simulink model "controller_test"  (R2021a)
settings: Solver=ode15s  StartTime=0.0  StopTime=0.75  FixedStep=0.00001  RelTol=1
InitFcn:
  | p_init;
  | p_init_wrist;
values from neighbouring files (symbols this model uses):
  a = 0    [p_init.m]
  a_w = 0    [p_init_wrist.m]
  b = 1/1.34e6    (= 7.46268656716e-07)    [p_init.m]
  b_w = 1/1.34e6    (= 7.46268656716e-07)    [p_init_wrist.m]
  comp_time = 0.000679456 * 1.25    (= 0.00084932)    [p_init.m]
  D_m = 0.00    (= 0)    [p_init.m]
  D_w = 0.00    (= 0)    [p_init_wrist.m]
  enc_res = 0.875 * pi/180    (= 0.015271630955)    [p_init.m]
  gear_ratio = 35    [p_init.m]
  gear_ratio_w = 36    [p_init_wrist.m]
  I_m = 0.00    (= 0)    [p_init.m]
  I_w = 0    [p_init_wrist.m]
  K_b = 1/(327*2*pi/60)    (= 0.0292027418517)    [p_init.m]
  K_b_w = 1/(1100*2*pi/60)    (= 0.0086811787141)    [p_init_wrist.m]
  K_m = 29.2 / 1000    (= 0.0292)    [p_init.m]
  K_m_w = 8.71 / 1000    (= 0.00871)    [p_init_wrist.m]
  K_p = 4.72e6/1.34e6    (= 3.5223880597)    [p_init.m]
  K_p_w = 4.72e6/1.34e6    (= 3.5223880597)    [p_init_wrist.m]
  L_term = 1.61 / 1000    (= 0.00161)    [p_init.m]
  L_term_w = 0.276 / 1000    (= 0.000276)    [p_init_wrist.m]
  P_m = 2.84    [p_init.m]
  P_w = 0.55    [p_init_wrist.m]
  R_term = 37.1    [p_init.m]
  R_term_w = 92.2    [p_init_wrist.m]
  v_max_amp = +V_nom    (= 24)    [p_init.m]
  v_max_amp_w = +V_nom_w    (= 12)    [p_init_wrist.m]
  v_min_amp = -V_nom    (= -24)    [p_init.m]
  v_min_amp_w = -V_nom_w    (= -12)    [p_init_wrist.m]
undefined symbols (not defined in the file or in its folder): f, fwd_kin_vect
libraries: simulink x6, pid_lib x3, instrumentlib x2
settings Model: Creator=Konstantin  LastModifiedBy=kossio
settings SolverCC: MaxOrder=3  ZeroCrossControl=DisableAll  AlgebraicLoopSolver=TrustRegion
settings DebuggingCC: SFMachineParentedDataDiag=warning

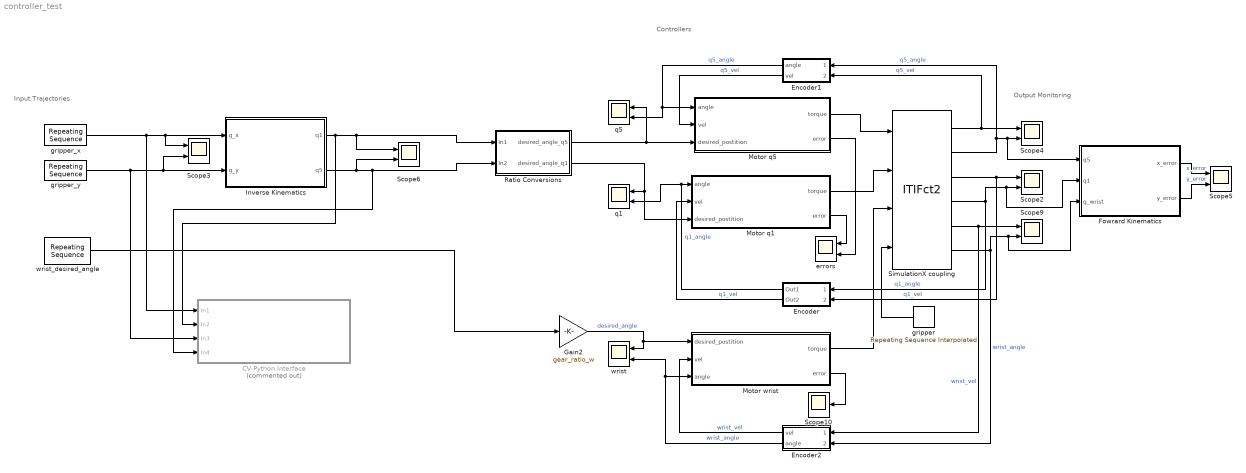
== system controller_test ==
  note: Output Monitoring
  note: Controllers
  note: Input Trajectories
  CV-Python Interface : Subsystem  Commented=on
  Encoder : Subsystem
  Encoder1 : Subsystem
  Encoder2 : Subsystem
  Fowrard Kinematics : Subsystem
  Gain2 : Gain  Gain=gear_ratio_w
  Inverse Kinematics : MATLAB Function  TreatAsAtomicUnit=on
  Motor q1 : Subsystem
  Motor q5 : Subsystem
  Motor wrist : Subsystem
  Ratio Conversions : Subsystem
  Scope10 : Scope
  Scope{2..6,9} (6 alike) : Scope  NumInputPorts=2
  SimulationX coupling : S-Function  FunctionName=ITIFct2  Parameters=ip, port, ts, nIn, nOut  SFunctionDeploymentMode=off  EnableBusSupport=off  mask{ip='localhost', port=4099, ts=0.001, nIn=4, nOut=6}
      mask prompts: ip "Address: ip"; port "Port Number: port [-]"; ts "Communication Step Size: ts [s]"; nIn "Input Vector Dimension (to SimulationX): nIn [-]"; nOut "Output Vector Dimension (from SimulationX): nOut [-]"
      mask help: Coupling Element
  errors : Scope  NumInputPorts=2
  gripper : simulink/Sources/Repeating Sequence Interpolated  OutValues=[0.2 0.2 10 0.2 10 0.2 10 0.2 0.2].'  TimeValues=[0 0.01 0.12 0.23 0.36 0.5 0.6 0.73 0.75].'  LookUpMeth=Use Input Below  tsamp=0.01  OutMin=[]  OutMax=[]  OutDataTypeStr=double  OutputDataTypeScalingMode=double  OutDataType=fixdt(0,8)  OutScaling=2^-10
  gripper_x : simulink/Sources/Repeating Sequence  rep_seq_t=time_vect  rep_seq_y=x_vect
  gripper_y : simulink/Sources/Repeating Sequence  rep_seq_t=time_vect  rep_seq_y=y_vect
  q1 : Scope  NumInputPorts=2
  q5 : Scope  NumInputPorts=2
  wrist : Scope  NumInputPorts=2
  wrist_desired_angle : simulink/Sources/Repeating Sequence  rep_seq_t=time_vect  rep_seq_y=wrist_angle
  wires:
  Inverse Kinematics/1(q1) -> CV-Python Interface/2(In2), Ratio Conversions/1(In1), Scope6/1
  Inverse Kinematics/2(q5) -> Scope6/2, Ratio Conversions/2(In2), CV-Python Interface/4(In4)
  gripper_y/1 -> CV-Python Interface/3(In3), Scope3/2, Inverse Kinematics/2(g_y)
  gripper_x/1 -> CV-Python Interface/1(In1), Inverse Kinematics/1(g_x), Scope3/1
  SimulationX coupling/1 -> Encoder1/2(2), Scope4/1  "q5_vel"
  SimulationX coupling/2 -> Fowrard Kinematics/1(q5), Scope4/2, Encoder1/1(1)  "q5_angle"
  SimulationX coupling/3 -> Encoder/2(2), Scope2/1  "q1_vel"
  SimulationX coupling/4 -> Encoder/1(1), Fowrard Kinematics/2(q1), Scope2/2  "q1_angle"
  Motor q1/2(error) -> errors/1
  Motor q5/2(error) -> errors/2
  SimulationX coupling/5 -> Encoder2/1(1), Scope9/1  "wrist_vel"
  SimulationX coupling/6 -> Fowrard Kinematics/3(q_wrist), Scope9/2, Encoder2/2(2)  "wrist_angle"
  Motor wrist/2(error) -> Scope10/1
  Motor wrist/1(torque) -> SimulationX coupling/3
  Gain2/1 -> wrist/1, Motor wrist/1(desired_postition)  "desired_angle"
  Motor q5/1(torque) -> SimulationX coupling/1
  Motor q1/1(torque) -> SimulationX coupling/2
  Encoder/1(Out1) -> q1/2, Motor q1/1(angle)  "q1_angle"
  Encoder/2(Out2) -> Motor q1/2(vel)  "q1_vel"
  Encoder1/1(angle) -> q5/2, Motor q5/1(angle)  "q5_angle"
  Encoder1/2(vel) -> Motor q5/2(vel)  "q5_vel"
  Ratio Conversions/2(desired_angle_q1) -> Motor q1/3(desired_postition), q1/1
  Ratio Conversions/1(desired_angle_q5) -> q5/1, Motor q5/3(desired_postition)
  Fowrard Kinematics/2(y_error) -> Scope5/2  "y_error"
  Fowrard Kinematics/1(x_error) -> Scope5/1  "x_error"
  wrist_desired_angle/1 -> Gain2/1
  Encoder2/1(vel) -> Motor wrist/2(vel)  "wrist_vel"
  Encoder2/2(angle) -> Motor wrist/3(angle), wrist/2  "wrist_angle"
  gripper/1 -> SimulationX coupling/4

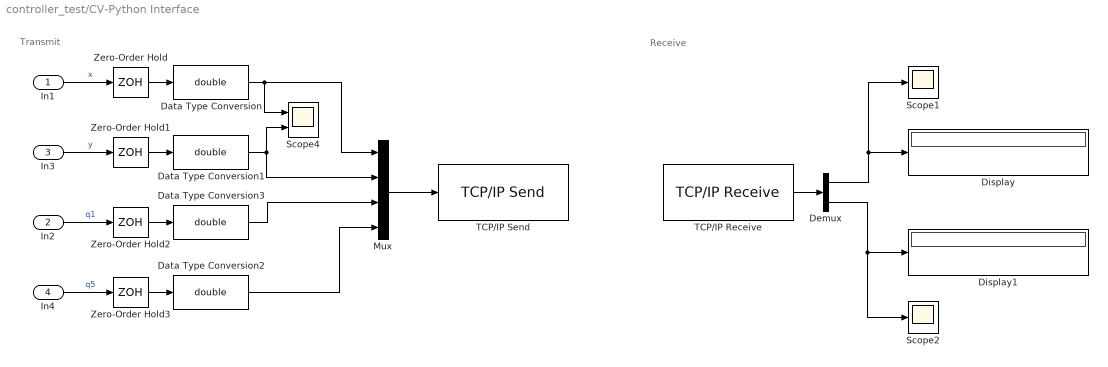
== system controller_test/CV-Python Interface ==
  note: Transmit
  note: Receive
  In1 : Inport
  In2 : Inport  Port=2
  In3 : Inport  Port=3
  In4 : Inport  Port=4
  Data Type Conversion{,1..3} (4 alike) : DataTypeConversion  OutDataTypeStr=double
  Demux : Demux  Outputs=2
  Display : Display
      settings: Format=decimal (Stored Integer)
  Display1 : Display
      settings: Format=decimal (Stored Integer)
  Mux : Mux
  Scope1 : Scope
  Scope2 : Scope
  Scope4 : Scope  NumInputPorts=2
  TCP/IP Receive : instrumentlib/TCP//IP Receive  Priority=1  Host=192.168.50.118  Port=10100  DataSize="[2  1]"  EnableBlockingMode=on  Timeout=10  SampleTime=0.01  DataType=double  ByteOrder=BigEndian  ASCIIFormatting=%f,  Terminator=LF
  TCP/IP Send : instrumentlib/TCP//IP Send  Priority=2  Host=192.168.50.118  Port=10100  EnableBlockingMode=on  Timeout=10  ByteOrder=BigEndian  TransferDelay=on
  Zero-Order Hold{,1..3} (4 alike) : ZeroOrderHold  SampleTime=0.01
  wires:
  Zero-Order Hold/1 -> Data Type Conversion/1
  TCP/IP Receive/1 -> Demux/1
  Demux/2 -> Scope2/1, Display1/1
  Zero-Order Hold2/1 -> Data Type Conversion3/1
  Data Type Conversion1/1 -> Scope4/2, Mux/2
  Zero-Order Hold1/1 -> Data Type Conversion1/1
  Demux/1 -> Display/1, Scope1/1
  Mux/1 -> TCP/IP Send/1
  Zero-Order Hold3/1 -> Data Type Conversion2/1
  Data Type Conversion/1 -> Scope4/1, Mux/1
  Data Type Conversion3/1 -> Mux/3
  Data Type Conversion2/1 -> Mux/4
  In4/1 -> Zero-Order Hold3/1  "q5"
  In2/1 -> Zero-Order Hold2/1  "q1"
  In1/1 -> Zero-Order Hold/1  "x"
  In3/1 -> Zero-Order Hold1/1  "y"

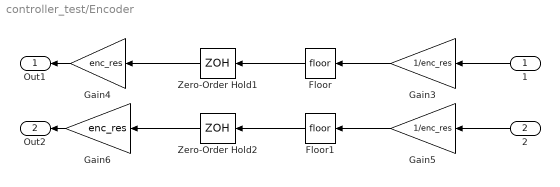
== system controller_test/Encoder ==
  1 : Inport
  2 : Inport  Port=2
  Floor : Rounding
  Floor1 : Rounding
  Gain3 : Gain  Gain=1/enc_res
  Gain4 : Gain  Gain=enc_res
  Gain5 : Gain  Gain=1/enc_res
  Gain6 : Gain  Gain=enc_res
  Zero-Order Hold1 : ZeroOrderHold  SampleTime=0.001
  Zero-Order Hold2 : ZeroOrderHold  SampleTime=0.001
  Out1 : Outport
  Out2 : Outport  Port=2
  wires:
  Zero-Order Hold2/1 -> Gain6/1
  Floor/1 -> Zero-Order Hold1/1
  Gain4/1 -> Out1/1
  Floor1/1 -> Zero-Order Hold2/1
  Gain6/1 -> Out2/1
  Gain5/1 -> Floor1/1
  Zero-Order Hold1/1 -> Gain4/1
  Gain3/1 -> Floor/1
  1/1 -> Gain3/1
  2/1 -> Gain5/1

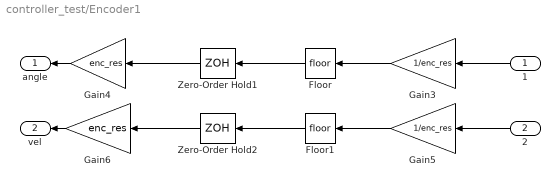
== system controller_test/Encoder1 ==
  1 : Inport
  2 : Inport  Port=2
  Floor : Rounding
  Floor1 : Rounding
  Gain3 : Gain  Gain=1/enc_res
  Gain4 : Gain  Gain=enc_res
  Gain5 : Gain  Gain=1/enc_res
  Gain6 : Gain  Gain=enc_res
  Zero-Order Hold1 : ZeroOrderHold  SampleTime=0.001
  Zero-Order Hold2 : ZeroOrderHold  SampleTime=0.001
  angle : Outport
  vel : Outport  Port=2
  wires:
  Zero-Order Hold2/1 -> Gain6/1
  Floor/1 -> Zero-Order Hold1/1
  Gain4/1 -> angle/1
  Floor1/1 -> Zero-Order Hold2/1
  Gain6/1 -> vel/1
  Gain5/1 -> Floor1/1
  Zero-Order Hold1/1 -> Gain4/1
  Gain3/1 -> Floor/1
  1/1 -> Gain3/1
  2/1 -> Gain5/1

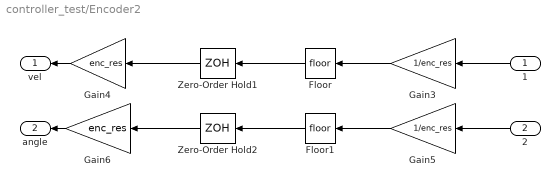
== system controller_test/Encoder2 ==
  1 : Inport
  2 : Inport  Port=2
  Floor : Rounding
  Floor1 : Rounding
  Gain3 : Gain  Gain=1/enc_res
  Gain4 : Gain  Gain=enc_res
  Gain5 : Gain  Gain=1/enc_res
  Gain6 : Gain  Gain=enc_res
  Zero-Order Hold1 : ZeroOrderHold  SampleTime=0.001
  Zero-Order Hold2 : ZeroOrderHold  SampleTime=0.001
  vel : Outport
  angle : Outport  Port=2
  wires:
  Zero-Order Hold2/1 -> Gain6/1
  Floor/1 -> Zero-Order Hold1/1
  Gain4/1 -> vel/1
  Floor1/1 -> Zero-Order Hold2/1
  Gain6/1 -> angle/1
  Gain5/1 -> Floor1/1
  Zero-Order Hold1/1 -> Gain4/1
  Gain3/1 -> Floor/1
  1/1 -> Gain3/1
  2/1 -> Gain5/1

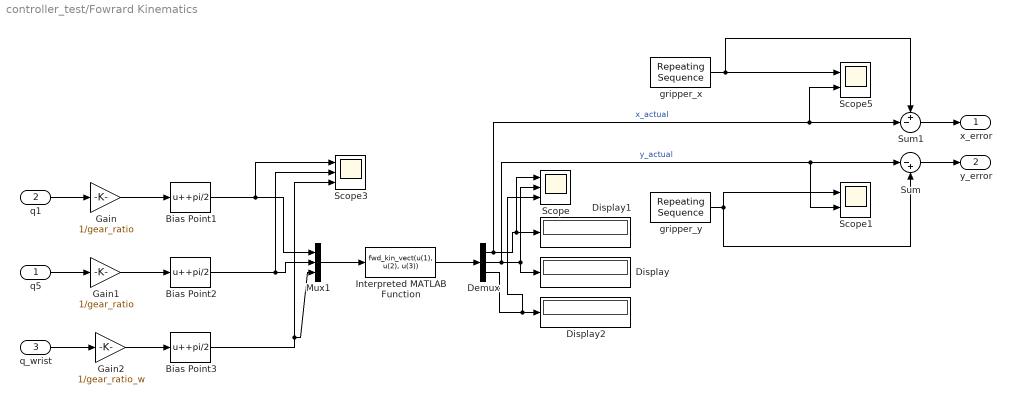
== system controller_test/Fowrard Kinematics ==
  q5 : Inport
  q1 : Inport  Port=2
  q_wrist : Inport  Port=3
  Bias Point1 : Bias  Bias=+pi/2
  Bias Point2 : Bias  Bias=+pi/2
  Bias Point3 : Bias  Bias=+pi/2
  Demux : Demux  Outputs=3
  Display : Display
  Display1 : Display
  Display2 : Display
  Gain : Gain  Gain=1/gear_ratio
  Gain1 : Gain  Gain=1/gear_ratio
  Gain2 : Gain  Gain=1/gear_ratio_w
  Interpreted MATLAB Function : MATLABFcn  MATLABFcn=fwd_kin_vect(u(1), u(2), u(3))  OutputDimensions=3
  Mux1 : Mux  Inputs=3
  Scope : Scope  NumInputPorts=3
  Scope1 : Scope  NumInputPorts=2
  Scope3 : Scope  NumInputPorts=3
  Scope5 : Scope  NumInputPorts=2
  Sum : Sum  Inputs=|-+
  Sum1 : Sum  Inputs=+-|
  gripper_x : simulink/Sources/Repeating Sequence  rep_seq_t=time_vect  rep_seq_y=x_vect
  gripper_y : simulink/Sources/Repeating Sequence  rep_seq_t=time_vect  rep_seq_y=y_vect
  x_error : Outport
  y_error : Outport  Port=2
  wires:
  Demux/3 -> Scope/3, Display2/1
  Interpreted MATLAB Function/1 -> Demux/1
  q5/1 -> Gain1/1
  Mux1/1 -> Interpreted MATLAB Function/1
  Demux/2 -> Scope1/2, Sum/1, Scope/2, Display/1  "y_actual"
  q1/1 -> Gain/1
  Demux/1 -> Scope5/2, Sum1/2, Scope/1, Display1/1  "x_actual"
  Gain/1 -> Bias Point1/1
  Gain1/1 -> Bias Point2/1
  gripper_y/1 -> Scope1/1, Sum/2
  gripper_x/1 -> Scope5/1, Sum1/1
  q_wrist/1 -> Gain2/1
  Gain2/1 -> Bias Point3/1
  Sum/1 -> y_error/1
  Sum1/1 -> x_error/1
  Bias Point1/1 -> Scope3/1, Mux1/1
  Bias Point2/1 -> Mux1/2, Scope3/2
  Bias Point3/1 -> Scope3/3, Mux1/3

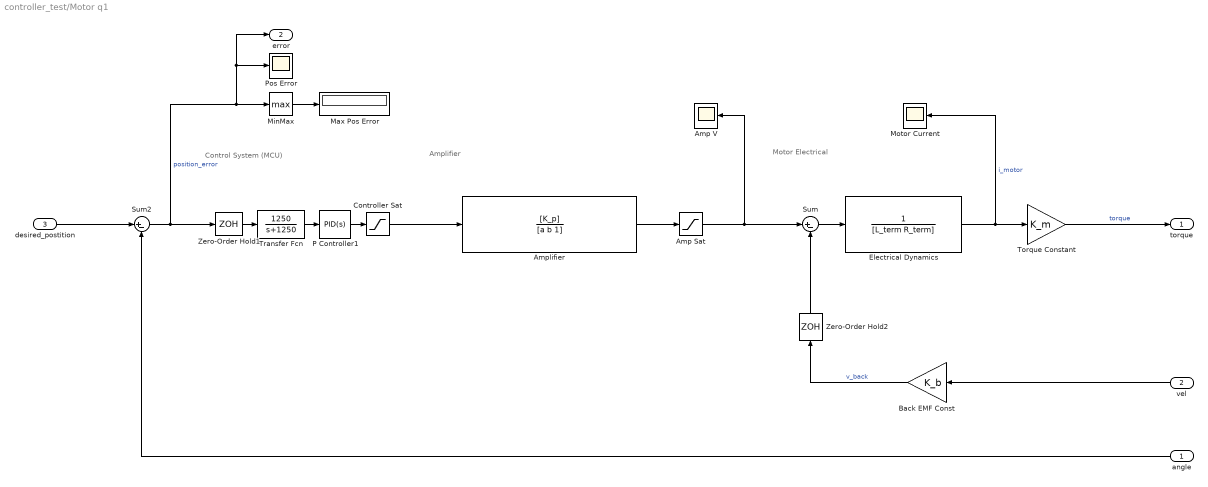
== system controller_test/Motor q1 ==
  note: Control System (MCU)
  note: Motor Electrical
  note: Amplifier
  angle : Inport
  vel : Inport  Port=2
  desired_postition : Inport  Port=3
  Amp Sat : Saturate  UpperLimit=v_max_amp  LowerLimit=v_min_amp
  Amp V : Scope
  Amplifier : TransferFcn  Numerator=[K_p]  Denominator=[a b 1]
  Back EMF Const : Gain  Gain=K_b
  Controller Sat : Saturate  UpperLimit=10  LowerLimit=-10
  Electrical Dynamics : TransferFcn  Denominator=[L_term R_term]
  Max Pos Error : Display
  MinMax : MinMax  Function=max
  Motor Current : Scope
  P Controller1 : pid_lib/PID Controller  Controller=PID  Form=Parallel  TimeDomain=Continuous-time  UseExternalTs=off  SampleTime=-1  IntegratorMethod=Forward Euler  FilterMethod=Forward Euler  ControllerParametersSource=internal  P=P_m  I=I_m  D=D_m  UseFilter=on  N=100  TunerSelectOption=Transfer Function Based (PID Tuner App)  InitialConditionSource=internal  InitialConditionForIntegrator=0  InitialConditionForFilter=0  DifferentiatorICPrevScaledInput=0  ExternalReset=none  TrackingMode=off  Kt=1  LimitOutput=off  SatLimitsSource=internal  UpperSaturationLimit=inf  LowerSaturationLimit=-inf  LinearizeAsGain=on  AntiWindupMode=none  Kb=1  POutMin=[]  POutMax=[]  IOutMin=[]  IOutMax=[]  DOutMin=[]  DOutMax=[]  NOutMin=[]  NOutMax=[]  SumOutMin=[]  SumOutMax=[]  SaturationOutMin=[]  SaturationOutMax=[]  PParamMin=[]  PParamMax=[]  IParamMin=[]  IParamMax=[]  DParamMin=[]  DParamMax=[]  NParamMin=[]  NParamMax=[]  KbParamMin=[]  KbParamMax=[]  KtParamMin=[]  KtParamMax=[]  KbOutMin=[]  KbOutMax=[]  KtOutMin=[]  KtOutMax=[]  IntegratorOutMin=[]  IntegratorOutMax=[]  FilterOutMin=[]  FilterOutMax=[]  SumI1OutMin=[]  SumI1OutMax=[]  SumI2OutMin=[]  SumI2OutMax=[]  SumI3OutMin=[]  SumI3OutMax=[]  SumI4OutMin=[]  SumI4OutMax=[]  SumDOutMin=[]  SumDOutMax=[]  DifferentiatorOutMin=[]  DifferentiatorOutMax=[]  FilterDiffOutCoefMin=[]  FilterDiffOutCoefMax=[]  ReciprocalOutMin=[]  ReciprocalOutMax=[]  SumDenOutMin=[]  SumDenOutMax=[]  SumNumOutMin=[]  SumNumOutMax=[]  DivideOutMin=[]  DivideOutMax=[]  UdiffTsProdOutMin=[]  UdiffTsProdOutMax=[]  NTsProdOutMin=[]  NTsProdOutMax=[]  UintegralTsProdOutMin=[]  UintegralTsProdOutMax=[]  UngainTsProdOutMin=[]  UngainTsProdOutMax=[]  IntegratorContinuousStateAttributes=''  IntegratorStateMustResolveToSignalObject=off  IntegratorRTWStateStorageClass=Auto  FilterContinuousStateAttributes=''  FilterStateMustResolveToSignalObject=off  FilterRTWStateStorageClass=Auto  ParallelPVariant=InternalParameters  IdealPVariant=Disabled  IVariant=InternalParameters  DVariant=InternalParameters  IntegratorVariant=Continuous  SatVariant=Disabled  AWVariant=Passthrough  PCopyVariant=Disabled  TRVariant=Disabled  FdbkBlocksVariant=Forward  IdealPFdbkVariant=Disabled  SatFdbkVariant=Disabled  DerivativeFilterVariant=ContFilter  NVariant=InternalParameters  NCopyVariant=Disabled  FilterICVariant=InternalICsFilter  IntegratorICVariant=InternalICs  ExternalResetVariant=Disabled  TRSumVariant=Passthrough  SumFdbkVariant=Disabled  SumVariant=Sum_PID  TsampFilterVariant=InternalTs  TsampNgainVariant=Passthrough  TsampIntegralVariant=Passthrough  ExternalSaturationOutDataTypeStr=Inherit: Same as second input
  Pos Error : Scope
  Sum : Sum  Inputs=|+-
  Sum2 : Sum  Inputs=|+-
  Torque Constant : Gain  Gain=K_m
  Transfer Fcn : TransferFcn  Numerator=[1250]  Denominator=[1 1250]
  Zero-Order Hold1 : ZeroOrderHold  SampleTime=comp_time
  Zero-Order Hold2 : ZeroOrderHold  SampleTime=comp_time
  torque : Outport
  error : Outport  Port=2
  wires:
  Sum2/1 -> Zero-Order Hold1/1, Pos Error/1, error/1, MinMax/1  "position_error"
  Amplifier/1 -> Amp Sat/1
  Amp Sat/1 -> Sum/1, Amp V/1
  P Controller1/1 -> Controller Sat/1
  Back EMF Const/1 -> Zero-Order Hold2/1  "v_back"
  Sum/1 -> Electrical Dynamics/1
  Electrical Dynamics/1 -> Motor Current/1, Torque Constant/1  "i_motor"
  Controller Sat/1 -> Amplifier/1
  MinMax/1 -> Max Pos Error/1
  Torque Constant/1 -> torque/1  "torque"
  angle/1 -> Sum2/2
  desired_postition/1 -> Sum2/1
  Zero-Order Hold1/1 -> Transfer Fcn/1
  vel/1 -> Back EMF Const/1
  Zero-Order Hold2/1 -> Sum/2
  Transfer Fcn/1 -> P Controller1/1

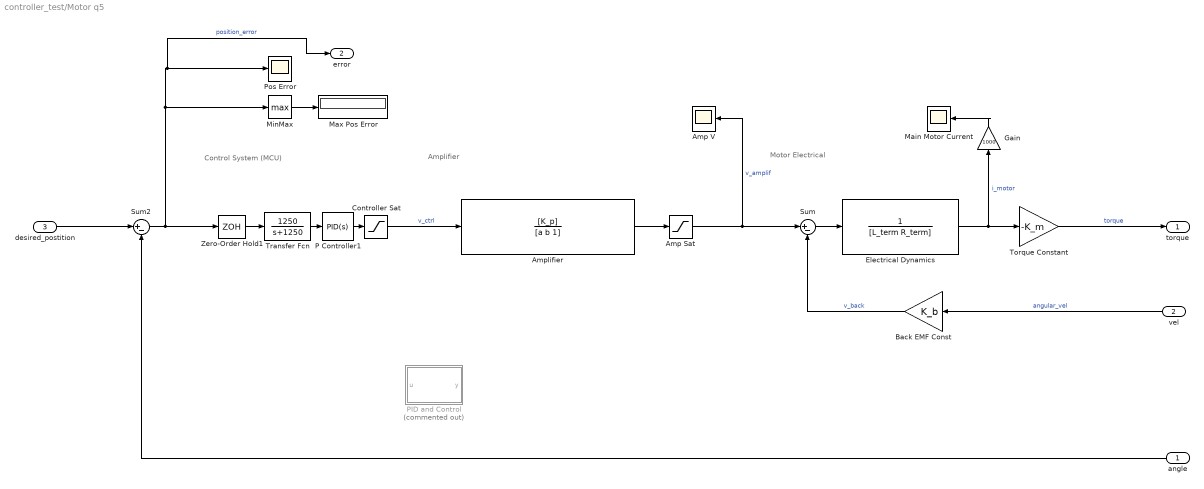
== system controller_test/Motor q5 ==
  note: Control System (MCU)
  note: Motor Electrical
  note: Amplifier
  angle : Inport
  vel : Inport  Port=2
  desired_postition : Inport  Port=3
  Amp Sat : Saturate  UpperLimit=v_max_amp  LowerLimit=v_min_amp
  Amp V : Scope
  Amplifier : TransferFcn  Numerator=[K_p]  Denominator=[a b 1]
  Back EMF Const : Gain  Gain=K_b
  Controller Sat : Saturate  UpperLimit=10  LowerLimit=-10
  Electrical Dynamics : TransferFcn  Denominator=[L_term R_term]
  Gain : Gain  Gain=1000
  Main Motor Current : Scope
  Max Pos Error : Display
  MinMax : MinMax  Function=max
  P Controller1 : pid_lib/PID Controller  Controller=PID  Form=Parallel  TimeDomain=Continuous-time  UseExternalTs=off  SampleTime=-1  IntegratorMethod=Forward Euler  FilterMethod=Forward Euler  ControllerParametersSource=internal  P=P_m  I=I_m  D=D_m  UseFilter=on  N=100  TunerSelectOption=Transfer Function Based (PID Tuner App)  InitialConditionSource=internal  InitialConditionForIntegrator=0  InitialConditionForFilter=0  DifferentiatorICPrevScaledInput=0  ExternalReset=none  TrackingMode=off  Kt=1  LimitOutput=off  SatLimitsSource=internal  UpperSaturationLimit=inf  LowerSaturationLimit=-inf  LinearizeAsGain=on  AntiWindupMode=none  Kb=1  POutMin=[]  POutMax=[]  IOutMin=[]  IOutMax=[]  DOutMin=[]  DOutMax=[]  NOutMin=[]  NOutMax=[]  SumOutMin=[]  SumOutMax=[]  SaturationOutMin=[]  SaturationOutMax=[]  PParamMin=[]  PParamMax=[]  IParamMin=[]  IParamMax=[]  DParamMin=[]  DParamMax=[]  NParamMin=[]  NParamMax=[]  KbParamMin=[]  KbParamMax=[]  KtParamMin=[]  KtParamMax=[]  KbOutMin=[]  KbOutMax=[]  KtOutMin=[]  KtOutMax=[]  IntegratorOutMin=[]  IntegratorOutMax=[]  FilterOutMin=[]  FilterOutMax=[]  SumI1OutMin=[]  SumI1OutMax=[]  SumI2OutMin=[]  SumI2OutMax=[]  SumI3OutMin=[]  SumI3OutMax=[]  SumI4OutMin=[]  SumI4OutMax=[]  SumDOutMin=[]  SumDOutMax=[]  DifferentiatorOutMin=[]  DifferentiatorOutMax=[]  FilterDiffOutCoefMin=[]  FilterDiffOutCoefMax=[]  ReciprocalOutMin=[]  ReciprocalOutMax=[]  SumDenOutMin=[]  SumDenOutMax=[]  SumNumOutMin=[]  SumNumOutMax=[]  DivideOutMin=[]  DivideOutMax=[]  UdiffTsProdOutMin=[]  UdiffTsProdOutMax=[]  NTsProdOutMin=[]  NTsProdOutMax=[]  UintegralTsProdOutMin=[]  UintegralTsProdOutMax=[]  UngainTsProdOutMin=[]  UngainTsProdOutMax=[]  IntegratorContinuousStateAttributes=''  IntegratorStateMustResolveToSignalObject=off  IntegratorRTWStateStorageClass=Auto  FilterContinuousStateAttributes=''  FilterStateMustResolveToSignalObject=off  FilterRTWStateStorageClass=Auto  ParallelPVariant=InternalParameters  IdealPVariant=Disabled  IVariant=InternalParameters  DVariant=InternalParameters  IntegratorVariant=Continuous  SatVariant=Disabled  AWVariant=Passthrough  PCopyVariant=Disabled  TRVariant=Disabled  FdbkBlocksVariant=Forward  IdealPFdbkVariant=Disabled  SatFdbkVariant=Disabled  DerivativeFilterVariant=ContFilter  NVariant=InternalParameters  NCopyVariant=Disabled  FilterICVariant=InternalICsFilter  IntegratorICVariant=InternalICs  ExternalResetVariant=Disabled  TRSumVariant=Passthrough  SumFdbkVariant=Disabled  SumVariant=Sum_PID  TsampFilterVariant=InternalTs  TsampNgainVariant=Passthrough  TsampIntegralVariant=Passthrough  ExternalSaturationOutDataTypeStr=Inherit: Same as second input
  PID and Control : MATLAB Function  Commented=on  TreatAsAtomicUnit=on
  Pos Error : Scope
  Sum : Sum  Inputs=|+-
  Sum2 : Sum  Inputs=|+-
  Torque Constant : Gain  Gain=-K_m
  Transfer Fcn : TransferFcn  Numerator=[1250]  Denominator=[1 1250]
  Zero-Order Hold1 : ZeroOrderHold  SampleTime=comp_time
  torque : Outport
  error : Outport  Port=2
  wires:
  Sum2/1 -> Zero-Order Hold1/1, MinMax/1, error/1, Pos Error/1  "position_error"
  Amp Sat/1 -> Sum/1, Amp V/1  "v_amplif"
  P Controller1/1 -> Controller Sat/1
  Back EMF Const/1 -> Sum/2  "v_back"
  Sum/1 -> Electrical Dynamics/1
  Electrical Dynamics/1 -> Torque Constant/1, Gain/1  "i_motor"
  Controller Sat/1 -> Amplifier/1  "v_ctrl"
  MinMax/1 -> Max Pos Error/1
  Torque Constant/1 -> torque/1  "torque"
  angle/1 -> Sum2/2
  vel/1 -> Back EMF Const/1  "angular_vel"
  desired_postition/1 -> Sum2/1
  Amplifier/1 -> Amp Sat/1
  Zero-Order Hold1/1 -> Transfer Fcn/1
  Gain/1 -> Main Motor Current/1
  Transfer Fcn/1 -> P Controller1/1

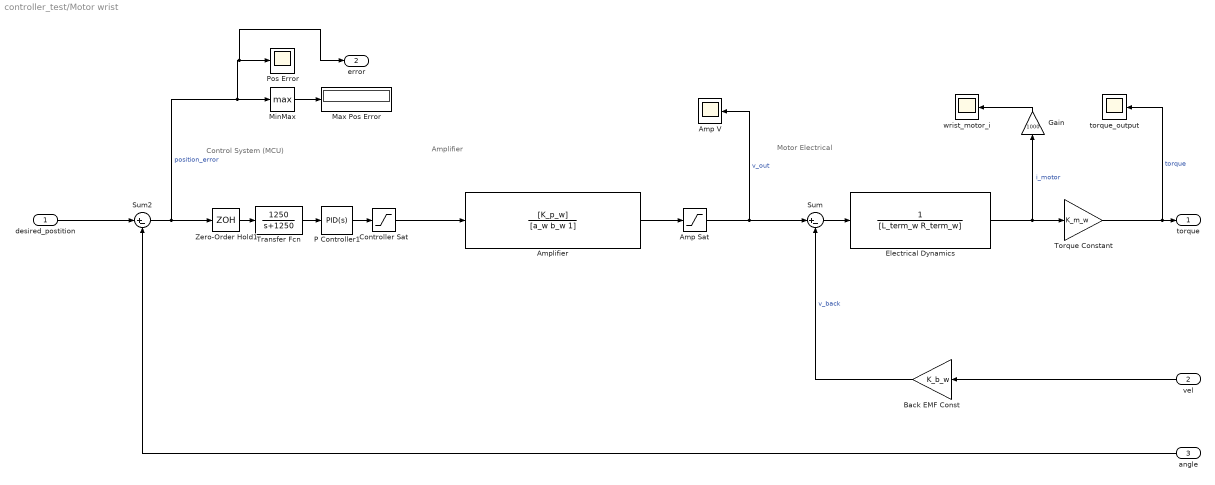
== system controller_test/Motor wrist ==
  note: Control System (MCU)
  note: Motor Electrical
  note: Amplifier
  desired_postition : Inport
  vel : Inport  Port=2
  angle : Inport  Port=3
  Amp Sat : Saturate  UpperLimit=v_max_amp_w  LowerLimit=v_min_amp_w
  Amp V : Scope
  Amplifier : TransferFcn  Numerator=[K_p_w]  Denominator=[a_w b_w 1]
  Back EMF Const : Gain  Gain=K_b_w
  Controller Sat : Saturate  UpperLimit=10  LowerLimit=-10
  Electrical Dynamics : TransferFcn  Denominator=[L_term_w R_term_w]
  Gain : Gain  Gain=1000
  Max Pos Error : Display
  MinMax : MinMax  Function=max
  P Controller1 : pid_lib/PID Controller  Controller=PID  Form=Parallel  TimeDomain=Continuous-time  UseExternalTs=off  SampleTime=-1  IntegratorMethod=Forward Euler  FilterMethod=Forward Euler  ControllerParametersSource=internal  P=P_w  I=I_w  D=D_w  UseFilter=on  N=100  TunerSelectOption=Transfer Function Based (PID Tuner App)  InitialConditionSource=internal  InitialConditionForIntegrator=0  InitialConditionForFilter=0  DifferentiatorICPrevScaledInput=0  ExternalReset=none  TrackingMode=off  Kt=1  LimitOutput=off  SatLimitsSource=internal  UpperSaturationLimit=inf  LowerSaturationLimit=-inf  LinearizeAsGain=on  AntiWindupMode=none  Kb=1  POutMin=[]  POutMax=[]  IOutMin=[]  IOutMax=[]  DOutMin=[]  DOutMax=[]  NOutMin=[]  NOutMax=[]  SumOutMin=[]  SumOutMax=[]  SaturationOutMin=[]  SaturationOutMax=[]  PParamMin=[]  PParamMax=[]  IParamMin=[]  IParamMax=[]  DParamMin=[]  DParamMax=[]  NParamMin=[]  NParamMax=[]  KbParamMin=[]  KbParamMax=[]  KtParamMin=[]  KtParamMax=[]  KbOutMin=[]  KbOutMax=[]  KtOutMin=[]  KtOutMax=[]  IntegratorOutMin=[]  IntegratorOutMax=[]  FilterOutMin=[]  FilterOutMax=[]  SumI1OutMin=[]  SumI1OutMax=[]  SumI2OutMin=[]  SumI2OutMax=[]  SumI3OutMin=[]  SumI3OutMax=[]  SumI4OutMin=[]  SumI4OutMax=[]  SumDOutMin=[]  SumDOutMax=[]  DifferentiatorOutMin=[]  DifferentiatorOutMax=[]  FilterDiffOutCoefMin=[]  FilterDiffOutCoefMax=[]  ReciprocalOutMin=[]  ReciprocalOutMax=[]  SumDenOutMin=[]  SumDenOutMax=[]  SumNumOutMin=[]  SumNumOutMax=[]  DivideOutMin=[]  DivideOutMax=[]  UdiffTsProdOutMin=[]  UdiffTsProdOutMax=[]  NTsProdOutMin=[]  NTsProdOutMax=[]  UintegralTsProdOutMin=[]  UintegralTsProdOutMax=[]  UngainTsProdOutMin=[]  UngainTsProdOutMax=[]  IntegratorContinuousStateAttributes=''  IntegratorStateMustResolveToSignalObject=off  IntegratorRTWStateStorageClass=Auto  FilterContinuousStateAttributes=''  FilterStateMustResolveToSignalObject=off  FilterRTWStateStorageClass=Auto  ParallelPVariant=InternalParameters  IdealPVariant=Disabled  IVariant=InternalParameters  DVariant=InternalParameters  IntegratorVariant=Continuous  SatVariant=Disabled  AWVariant=Passthrough  PCopyVariant=Disabled  TRVariant=Disabled  FdbkBlocksVariant=Forward  IdealPFdbkVariant=Disabled  SatFdbkVariant=Disabled  DerivativeFilterVariant=ContFilter  NVariant=InternalParameters  NCopyVariant=Disabled  FilterICVariant=InternalICsFilter  IntegratorICVariant=InternalICs  ExternalResetVariant=Disabled  TRSumVariant=Passthrough  SumFdbkVariant=Disabled  SumVariant=Sum_PID  TsampFilterVariant=InternalTs  TsampNgainVariant=Passthrough  TsampIntegralVariant=Passthrough  ExternalSaturationOutDataTypeStr=Inherit: Same as second input
  Pos Error : Scope
  Sum : Sum  Inputs=|+-
  Sum2 : Sum  Inputs=|+-
  Torque Constant : Gain  Gain=K_m_w
  Transfer Fcn : TransferFcn  Numerator=[1250]  Denominator=[1 1250]
  Zero-Order Hold1 : ZeroOrderHold  SampleTime=comp_time
  torque_output : Scope
  wrist_motor_i : Scope
  torque : Outport
  error : Outport  Port=2
  wires:
  Sum2/1 -> Zero-Order Hold1/1, error/1, Pos Error/1, MinMax/1  "position_error"
  Amplifier/1 -> Amp Sat/1
  Amp Sat/1 -> Sum/1, Amp V/1  "v_out"
  P Controller1/1 -> Controller Sat/1
  Back EMF Const/1 -> Sum/2  "v_back"
  Sum/1 -> Electrical Dynamics/1
  Electrical Dynamics/1 -> Torque Constant/1, Gain/1  "i_motor"
  Controller Sat/1 -> Amplifier/1
  MinMax/1 -> Max Pos Error/1
  Torque Constant/1 -> torque_output/1, torque/1  "torque"
  angle/1 -> Sum2/2
  vel/1 -> Back EMF Const/1
  desired_postition/1 -> Sum2/1
  Zero-Order Hold1/1 -> Transfer Fcn/1
  Transfer Fcn/1 -> P Controller1/1
  Gain/1 -> wrist_motor_i/1

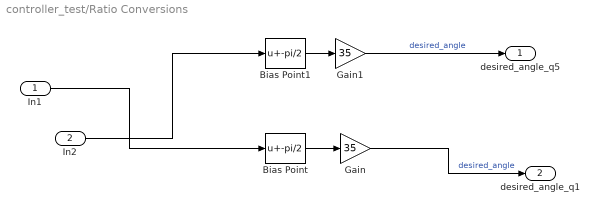
== system controller_test/Ratio Conversions ==
  In1 : Inport
  In2 : Inport  Port=2
  Bias Point : Bias  Bias=-pi/2
  Bias Point1 : Bias  Bias=-pi/2
  Gain : Gain  Gain=35
  Gain1 : Gain  Gain=35
  desired_angle_q5 : Outport
  desired_angle_q1 : Outport  Port=2
  wires:
  Bias Point/1 -> Gain/1
  Gain/1 -> desired_angle_q1/1  "desired_angle"
  Bias Point1/1 -> Gain1/1
  Gain1/1 -> desired_angle_q5/1  "desired_angle"
  In2/1 -> Bias Point1/1
  In1/1 -> Bias Point/1

== matlab function controller_test/Motor q5/PID and Control ==
  data: u input; y output
function y = fcn(u)
global P_m;

y = P_m * u;

== matlab function controller_test/Inverse Kinematics ==
  data: g_x input; q1 output; g_y input; q5 output
function [q1, q5] = inv_kin(g_x, g_y)
% Calculates inverse kinematics of robot
% @param x position of gripper center
% @param y position of gripper center
% @return q1, q2 of motors

    l1 = 6.5; l4 = l1;     % arms attached to motors
    l2 = 8.5; l3 = l2;     % arms attached to gripper
    l5 = 4;                % motor spacing, 5th link
    xg = 0;                % x offset from q3 to gripper center 
    yg = 3.5;                % y offset from q3 to gripper center 
    
    % calculate position of wrist
    x = g_x - xg;
    y = g_y - yg;
    
    % find vector lengths to wrist joint
    p = sqrt(x^2 + y^2);
    r = sqrt((x+l5)^2 + y^2);
    
    % calculate angles to p and r vectors from x-axis
    alpha = acos(x/p);
    beta = acos((x+l5)/r);
    
    % use law of cosines to find inner angle of triangles
    q1_p = acos((p^2 + l1^2 - l2^2) / (2*p*l1));
    q5_p = acos((r^2 + l4^2 - l3^2) / (2*r*l4));
    
    % find q1 and q5 motor angles
    q1 = alpha - q1_p;
    q5 = beta + q5_p;
    
end
